simulink library "jcw"  (Simulink 8.1)
settings: Solver=ode45  StartTime=0.0  StopTime=10.0  RelTol=1e-3
libraries: ftc x1, fac x1, fdc x1, fen x1, foc x1, fro x1, fsr x1
settings Model: Creator=xsellart  LastModifiedBy=AT015555

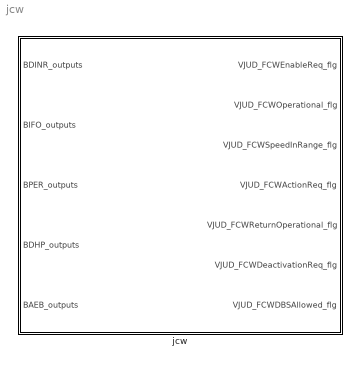
== system jcw ==
  jcw : Subsystem

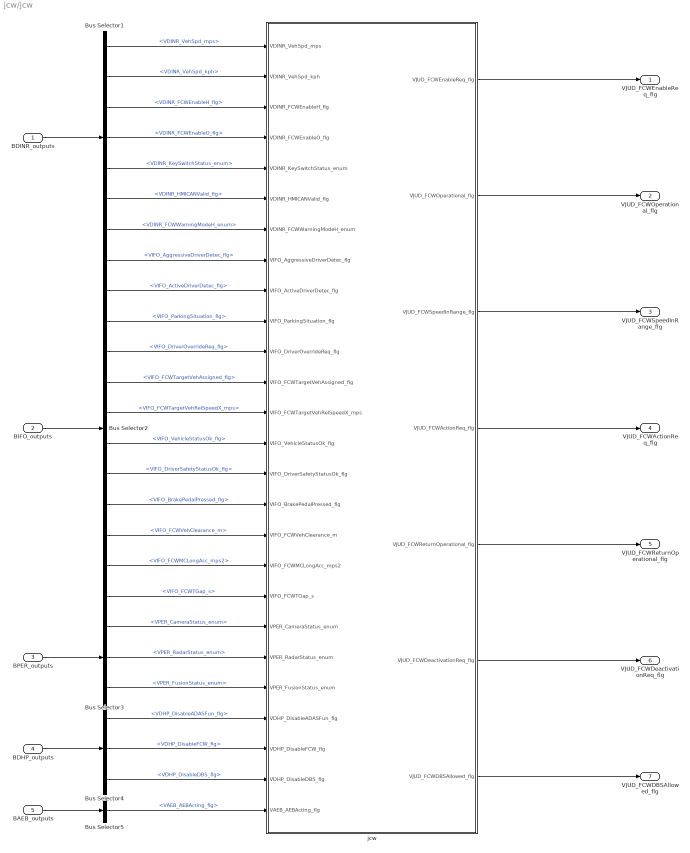
== system jcw/jcw ==
  BDINR_outputs : Inport  OutDataTypeStr=Bus: BDINR_outputs
  BIFO_outputs : Inport  Port=2  OutDataTypeStr=Bus: BIFO_outputs
  BPER_outputs : Inport  Port=3  OutDataTypeStr=Bus: BPER_outputs
  BDHP_outputs : Inport  Port=4  OutDataTypeStr=Bus: BDHP_outputs
  BAEB_outputs : Inport  Port=5  OutDataTypeStr=Bus: BAEB_outputs
  Bus Selector1 : BusSelector  OutputSignals=VDINR_VehSpd_mps,VDINR_VehSpd_kph,VDINR_FCWEnableH_flg,VDINR_FCWEnableO_flg,VDINR_KeySwitchStatus_enum,VDINR_HMICANValid_flg,VDINR_FCWWarningModeH_enum
  Bus Selector2 : BusSelector  OutputSignals=VIFO_AggressiveDriverDetec_flg,VIFO_ActiveDriverDetec_flg,VIFO_ParkingSituation_flg,VIFO_DriverOverrideReq_flg,VIFO_FCWTargetVehAssigned_flg,VIFO_FCWTargetVehRelSpeedX_mps,VIFO_VehicleStatusOk_flg,VIFO_DriverSafetyStatusOk_flg,VIFO_BrakePedalPressed_flg,VIFO_FCWVehClearance_m,VIFO_FCWMCLongAcc_mps2,VIFO_FCWTGap_s
  Bus Selector3 : BusSelector  OutputSignals=VPER_CameraStatus_enum,VPER_RadarStatus_enum,VPER_FusionStatus_enum
  Bus Selector4 : BusSelector  OutputSignals=VDHP_DisableADASFun_flg,VDHP_DisableFCW_flg,VDHP_DisableDBS_flg
  Bus Selector5 : BusSelector  OutputSignals=VAEB_AEBActing_flg
  jcw : Subsystem
  VJUD_FCWEnableReq_flg : Outport
  VJUD_FCWOperational_flg : Outport  Port=2
  VJUD_FCWSpeedInRange_flg : Outport  Port=3
  VJUD_FCWActionReq_flg : Outport  Port=4
  VJUD_FCWReturnOperational_flg : Outport  Port=5
  VJUD_FCWDeactivationReq_flg : Outport  Port=6
  VJUD_FCWDBSAllowed_flg : Outport  Port=7
  wires:
  Bus Selector2/11 -> jcw/18(VIFO_FCWMCLongAcc_mps2)  "<VIFO_FCWMCLongAcc_mps2>"
  Bus Selector1/1 -> jcw/1(VDINR_VehSpd_mps)  "<VDINR_VehSpd_mps>"
  Bus Selector2/10 -> jcw/17(VIFO_FCWVehClearance_m)  "<VIFO_FCWVehClearance_m>"
  jcw/5(VJUD_FCWReturnOperational_flg) -> VJUD_FCWReturnOperational_flg/1
  Bus Selector5/1 -> jcw/26(VAEB_AEBActing_flg)  "<VAEB_AEBActing_flg>"
  BAEB_outputs/1 -> Bus Selector5/1
  Bus Selector1/4 -> jcw/4(VDINR_FCWEnableO_flg)  "<VDINR_FCWEnableO_flg>"
  Bus Selector1/3 -> jcw/3(VDINR_FCWEnableH_flg)  "<VDINR_FCWEnableH_flg>"
  Bus Selector4/3 -> jcw/25(VDHP_DisableDBS_flg)  "<VDHP_DisableDBS_flg>"
  Bus Selector2/9 -> jcw/16(VIFO_BrakePedalPressed_flg)  "<VIFO_BrakePedalPressed_flg>"
  Bus Selector4/1 -> jcw/23(VDHP_DisableADASFun_flg)  "<VDHP_DisableADASFun_flg>"
  Bus Selector4/2 -> jcw/24(VDHP_DisableFCW_flg)  "<VDHP_DisableFCW_flg>"
  BDHP_outputs/1 -> Bus Selector4/1
  Bus Selector1/2 -> jcw/2(VDINR_VehSpd_kph)  "<VDINR_VehSpd_kph>"
  Bus Selector3/3 -> jcw/22(VPER_FusionStatus_enum)  "<VPER_FusionStatus_enum>"
  Bus Selector1/6 -> jcw/6(VDINR_HMICANValid_flg)  "<VDINR_HMICANValid_flg>"
  Bus Selector3/1 -> jcw/20(VPER_CameraStatus_enum)  "<VPER_CameraStatus_enum>"
  Bus Selector1/5 -> jcw/5(VDINR_KeySwitchStatus_enum)  "<VDINR_KeySwitchStatus_enum>"
  Bus Selector3/2 -> jcw/21(VPER_RadarStatus_enum)  "<VPER_RadarStatus_enum>"
  Bus Selector2/4 -> jcw/11(VIFO_DriverOverrideReq_flg)  "<VIFO_DriverOverrideReq_flg>"
  Bus Selector2/1 -> jcw/8(VIFO_AggressiveDriverDetec_flg)  "<VIFO_AggressiveDriverDetec_flg>"
  Bus Selector1/7 -> jcw/7(VDINR_FCWWarningModeH_enum)  "<VDINR_FCWWarningModeH_enum>"
  Bus Selector2/3 -> jcw/10(VIFO_ParkingSituation_flg)  "<VIFO_ParkingSituation_flg>"
  Bus Selector2/2 -> jcw/9(VIFO_ActiveDriverDetec_flg)  "<VIFO_ActiveDriverDetec_flg>"
  Bus Selector2/6 -> jcw/13(VIFO_FCWTargetVehRelSpeedX_mps)  "<VIFO_FCWTargetVehRelSpeedX_mps>"
  Bus Selector2/5 -> jcw/12(VIFO_FCWTargetVehAssigned_flg)  "<VIFO_FCWTargetVehAssigned_flg>"
  BIFO_outputs/1 -> Bus Selector2/1
  BDINR_outputs/1 -> Bus Selector1/1
  Bus Selector2/8 -> jcw/15(VIFO_DriverSafetyStatusOk_flg)  "<VIFO_DriverSafetyStatusOk_flg>"
  Bus Selector2/7 -> jcw/14(VIFO_VehicleStatusOk_flg)  "<VIFO_VehicleStatusOk_flg>"
  BPER_outputs/1 -> Bus Selector3/1
  jcw/1(VJUD_FCWEnableReq_flg) -> VJUD_FCWEnableReq_flg/1
  jcw/7(VJUD_FCWDBSAllowed_flg) -> VJUD_FCWDBSAllowed_flg/1
  jcw/4(VJUD_FCWActionReq_flg) -> VJUD_FCWActionReq_flg/1
  jcw/2(VJUD_FCWOperational_flg) -> VJUD_FCWOperational_flg/1
  jcw/6(VJUD_FCWDeactivationReq_flg) -> VJUD_FCWDeactivationReq_flg/1
  jcw/3(VJUD_FCWSpeedInRange_flg) -> VJUD_FCWSpeedInRange_flg/1
  Bus Selector2/12 -> jcw/19(VIFO_FCWTGap_s)  "<VIFO_FCWTGap_s>"

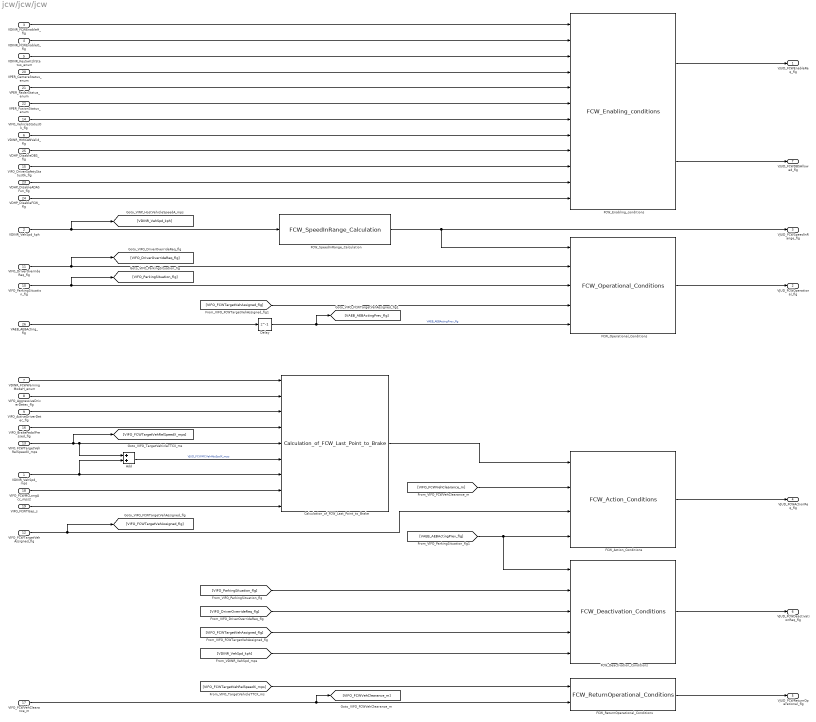
== system jcw/jcw/jcw ==
  VDINR_VehSpd_mps : Inport
  VDINR_VehSpd_kph : Inport  Port=2
  VDINR_FCWEnableH_flg : Inport  Port=3
  VDINR_FCWEnableO_flg : Inport  Port=4
  VDINR_KeySwitchStatus_enum : Inport  Port=5
  VDINR_HMICANValid_flg : Inport  Port=6
  VDINR_FCWWarningModeH_enum : Inport  Port=7
  VIFO_AggressiveDriverDetec_flg : Inport  Port=8
  VIFO_ActiveDriverDetec_flg : Inport  Port=9
  VIFO_ParkingSituation_flg : Inport  Port=10
  VIFO_DriverOverrideReq_flg : Inport  Port=11
  VIFO_FCWTargetVehAssigned_flg : Inport  Port=12
  VIFO_FCWTargetVehRelSpeedX_mps : Inport  Port=13
  VIFO_VehicleStatusOk_flg : Inport  Port=14
  VIFO_DriverSafetyStatusOk_flg : Inport  Port=15
  VIFO_BrakePedalPressed_flg : Inport  Port=16
  VIFO_FCWVehClearance_m : Inport  Port=17
  VIFO_FCWMCLongAcc_mps2 : Inport  Port=18
  VIFO_FCWTGap_s : Inport  Port=19
  VPER_CameraStatus_enum : Inport  Port=20
  VPER_RadarStatus_enum : Inport  Port=21
  VPER_FusionStatus_enum : Inport  Port=22
  VDHP_DisableADASFun_flg : Inport  Port=23
  VDHP_DisableFCW_flg : Inport  Port=24
  VDHP_DisableDBS_flg : Inport  Port=25
  VAEB_AEBActing_flg : Inport  Port=26
  Add : Sum
  Calculation_of_FCW_Last_Point_to_Brake : ftc/Calculation_of_FCW_Last_Point_to_Brake
  Delay : Delay  DelayLength=1  InitialCondition=0
  FCW_Action_Conditions : fac/FCW_Action_Conditions
  FCW_Deactivation_Conditions : fdc/FCW_Deactivation_Conditions
  FCW_Enabling_conditions : fen/FCW_Enabling_conditions
  FCW_Operational_Conditions : foc/FCW_Operational_Conditions
  FCW_ReturnOperational_Conditions : fro/FCW_ReturnOperational_Conditions
  FCW_SpeedInRange_Calculation : fsr/FCW_SpeedInRange_Calculation
  VJUD_FCWEnableReq_flg : Outport
  VJUD_FCWOperational_flg : Outport  Port=2
  VJUD_FCWSpeedInRange_flg : Outport  Port=3
  VJUD_FCWActionReq_flg : Outport  Port=4
  VJUD_FCWReturnOperational_flg : Outport  Port=5
  VJUD_FCWDeactivationReq_flg : Outport  Port=6
  VJUD_FCWDBSAllowed_flg : Outport  Port=7
  wires:
  [VIFO_FCWVehClearance_m] -> FCW_Action_Conditions/2
  Calculation_of_FCW_Last_Point_to_Brake/1 -> FCW_Action_Conditions/1
  Add/1 -> Calculation_of_FCW_Last_Point_to_Brake/6  "VJUD_FCWMCVehAbsSpdX_mps"
  VDINR_VehSpd_mps/1 -> Calculation_of_FCW_Last_Point_to_Brake/7, Add/2
  VIFO_FCWMCLongAcc_mps2/1 -> Calculation_of_FCW_Last_Point_to_Brake/8
  VDINR_FCWWarningModeH_enum/1 -> Calculation_of_FCW_Last_Point_to_Brake/1
  VIFO_FCWVehClearance_m/1 -> FCW_ReturnOperational_Conditions/2, [VIFO_FCWVehClearance_m]
  [VIFO_FCWTargetVehRelSpeedX_mps] -> FCW_ReturnOperational_Conditions/1
  FCW_ReturnOperational_Conditions/1 -> VJUD_FCWReturnOperational_flg/1
  Delay/1 -> FCW_Operational_Conditions/5, [VAEB_AEBActingPrev_flg]  "VAEB_AEBActingPrev_flg"
  [VDINR_VehSpd_kph] -> FCW_Deactivation_Conditions/5
  [VAEB_AEBActingPrev_flg] -> FCW_Action_Conditions/4, FCW_Deactivation_Conditions/1
  VIFO_BrakePedalPressed_flg/1 -> Calculation_of_FCW_Last_Point_to_Brake/4
  VDHP_DisableADASFun_flg/1 -> FCW_Enabling_conditions/11
  VDHP_DisableDBS_flg/1 -> FCW_Enabling_conditions/9
  VDHP_DisableFCW_flg/1 -> FCW_Enabling_conditions/12
  [VIFO_FCWTargetVehAssigned_flg] -> FCW_Operational_Conditions/4
  FCW_Enabling_conditions/1 -> VJUD_FCWEnableReq_flg/1
  VIFO_FCWTargetVehAssigned_flg/1 -> FCW_Action_Conditions/3, [VIFO_FCWTargetVehAssigned_flg]
  VIFO_AggressiveDriverDetec_flg/1 -> Calculation_of_FCW_Last_Point_to_Brake/2
  VIFO_ActiveDriverDetec_flg/1 -> Calculation_of_FCW_Last_Point_to_Brake/3
  FCW_Operational_Conditions/1 -> VJUD_FCWOperational_flg/1
  FCW_Action_Conditions/1 -> VJUD_FCWActionReq_flg/1
  [VIFO_ParkingSituation_flg] -> FCW_Deactivation_Conditions/2
  [VIFO_DriverOverrideReq_flg] -> FCW_Deactivation_Conditions/3
  FCW_Deactivation_Conditions/1 -> VJUD_FCWDeactivationReq_flg/1
  FCW_SpeedInRange_Calculation/1 -> VJUD_FCWSpeedInRange_flg/1, FCW_Operational_Conditions/1
  VAEB_AEBActing_flg/1 -> Delay/1
  [VIFO_FCWTargetVehAssigned_flg] -> FCW_Deactivation_Conditions/4
  VDINR_FCWEnableH_flg/1 -> FCW_Enabling_conditions/1
  VDINR_FCWEnableO_flg/1 -> FCW_Enabling_conditions/2
  VDINR_KeySwitchStatus_enum/1 -> FCW_Enabling_conditions/3
  VIFO_DriverSafetyStatusOk_flg/1 -> FCW_Enabling_conditions/10
  VPER_CameraStatus_enum/1 -> FCW_Enabling_conditions/4
  VIFO_VehicleStatusOk_flg/1 -> FCW_Enabling_conditions/7
  VDINR_HMICANValid_flg/1 -> FCW_Enabling_conditions/8
  VPER_FusionStatus_enum/1 -> FCW_Enabling_conditions/6
  VPER_RadarStatus_enum/1 -> FCW_Enabling_conditions/5
  FCW_Enabling_conditions/2 -> VJUD_FCWDBSAllowed_flg/1
  VDINR_VehSpd_kph/1 -> FCW_SpeedInRange_Calculation/1, [VDINR_VehSpd_kph]
  VIFO_DriverOverrideReq_flg/1 -> [VIFO_DriverOverrideReq_flg], FCW_Operational_Conditions/2
  VIFO_ParkingSituation_flg/1 -> FCW_Operational_Conditions/3, [VIFO_ParkingSituation_flg]
  VIFO_FCWTargetVehRelSpeedX_mps/1 -> [VIFO_FCWTargetVehRelSpeedX_mps], Add/1, Calculation_of_FCW_Last_Point_to_Brake/5
  VIFO_FCWTGap_s/1 -> Calculation_of_FCW_Last_Point_to_Brake/9
